simulink model "Pokus08_Matlab_Function"  (Simulink 8.1)
settings: Solver=FixedStepDiscrete  StartTime=0.0  StopTime=10.0  FixedStep=1  RelTol=1e-3
settings Model: Creator=uzivatel  LastModifiedBy=uzivatel
settings DataIOCC: SignalLoggingSaveFormat=Dataset
settings OptimizationCC: ExpressionDepthLimit=128
settings DebuggingCC: FcnCallInpInsideContextMsg=EnableAllAsError
settings GRTTargetCC: CombineOutputUpdateFcns=on  GRTInterface=off

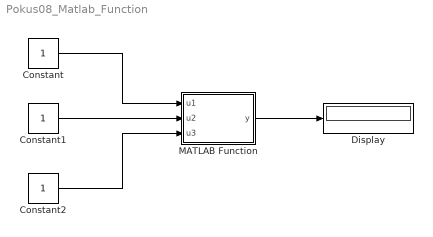
== system Pokus08_Matlab_Function ==
  Constant : Constant  OutDataTypeStr=uint8
  Constant1 : Constant  OutDataTypeStr=uint8
  Constant2 : Constant  OutDataTypeStr=uint8
  Display : Display
  MATLAB Function : MATLAB Function  TreatAsAtomicUnit=on
  wires:
  Constant/1 -> MATLAB Function/1(u1)
  Constant1/1 -> MATLAB Function/2(u2)
  Constant2/1 -> MATLAB Function/3(u3)
  MATLAB Function/1(y) -> Display/1

== matlab function MATLAB Function ==
  data: u1 input double; y output double; u2 input double; u3 input double
function y = fcn(u1, u2, u3)

y = u1 + u2 + u3;
end
